simulink model "sim_linear_control_y"  (R2018a)
settings: Solver=ode3  StartTime=0.0  StopTime=20  FixedStep=0.001  RelTol=1e-3
values from neighbouring files (symbols this model uses):
  A = [-(Cf+Cr)/(m*Vx)  -(a*Cf-b*Cr)/(m*Vx)-Vx ... (first row only)    [lin_control_pos_v1.m]    (also in lin_control_y.m)
  B = [Cf/m; a*Cf/Iz]    [lin_control_pos_v1.m]    (also in lin_control_y.m)
  C = Col(3,:)    [lin_control_pos_v1.m]    (also in lin_control_y.m)
  CA = C*Aol    [lin_control_pos_v1.m]    (also in lin_control_y.m)
  g = 9.81    [lin_control_pos_v1.m]    (also in lin_control_y.m)
  intgA = zeros(2,2)    [lin_control_y.m]
  intgB = eye(2)    [lin_control_y.m]
  intgC = eye(2)    [lin_control_y.m]
  intgD = zeros(2,2)    [lin_control_y.m]
  invCB = pinv(C*Bol)    [lin_control_pos_v1.m]    (also in lin_control_y.m)
  K_ay = 8    [lin_control_pos_v1.m]    (also in lin_control_y.m = 4)
  K_v = 1    [lin_control_y.m]
  loop = 1    [lin_control_y.m]
  rho = 1/R    (= 0.05)    [lin_control_pos_v1.m]    (also in lin_control_y.m)
  Vx = 10/3.6    (= 2.77777777778)    [lin_control_pos_v1.m]    (also in lin_control_y.m)
  w = 10    [lin_control_pos_v1.m]    (also in lin_control_y.m)
settings Model: Creator=E183308  LastModifiedBy=E183308

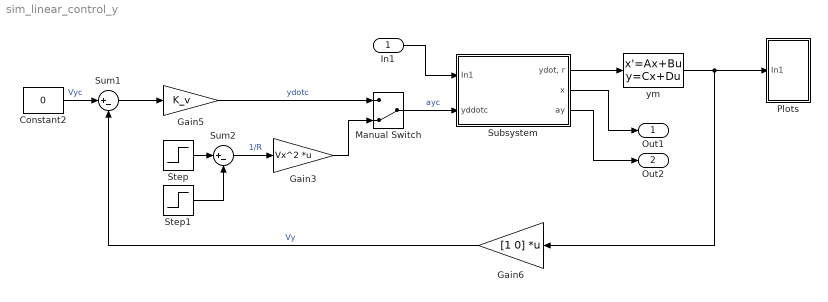
== system sim_linear_control_y ==
  In1 : Inport
  Constant2 : Constant  Value=0
  Gain3 : Gain  Gain=Vx^2  Multiplication=Matrix(K*u)
  Gain5 : Gain  Gain=K_v
  Gain6 : Gain  Gain=[1 0]  Multiplication=Matrix(K*u)
  Manual Switch : ManualSwitch  CurrentSetting=0
  Plots : Subsystem
  Step : Step  After=rho  SampleTime=0
  Step1 : Step  Time=10  After=rho  SampleTime=0
  Subsystem : Subsystem
  Sum1 : Sum  Inputs=|+-
  Sum2 : Sum  Inputs=|+-
  ym : StateSpace  A=intgA  B=intgB  C=intgC  D=intgD  InitialCondition=0
  Out1 : Outport
  Out2 : Outport  Port=2
  wires:
  Gain5/1 -> Manual Switch/1  "ydotc"
  Sum1/1 -> Gain5/1
  Gain6/1 -> Sum1/2  "Vy"
  In1/1 -> Subsystem/1(In1)
  Manual Switch/1 -> Subsystem/2(yddotc)  "ayc"
  ym/1 -> Gain6/1, Plots/1(In1)
  Subsystem/2(x) -> Out1/1
  Subsystem/1("ydot, r") -> ym/1
  Subsystem/3(ay) -> Out2/1
  Constant2/1 -> Sum1/1  "Vyc"
  Step1/1 -> Sum2/2
  Step/1 -> Sum2/1
  Sum2/1 -> Gain3/1  "1/R"
  Gain3/1 -> Manual Switch/2

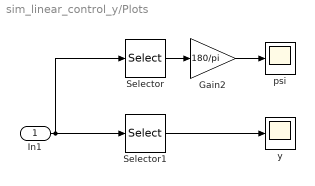
== system sim_linear_control_y/Plots ==
  In1 : Inport
  Gain2 : Gain  Gain=180/pi
  Selector : Selector  InputPortWidth=2  IndexOptions=Index vector (dialog)  Indices=2  OutputSizes=1
  Selector1 : Selector  InputPortWidth=2  IndexOptions=Index vector (dialog)  Indices=1  OutputSizes=1
  psi : Scope
  y : Scope
  wires:
  Gain2/1 -> psi/1
  In1/1 -> Selector1/1, Selector/1
  Selector/1 -> Gain2/1
  Selector1/1 -> y/1

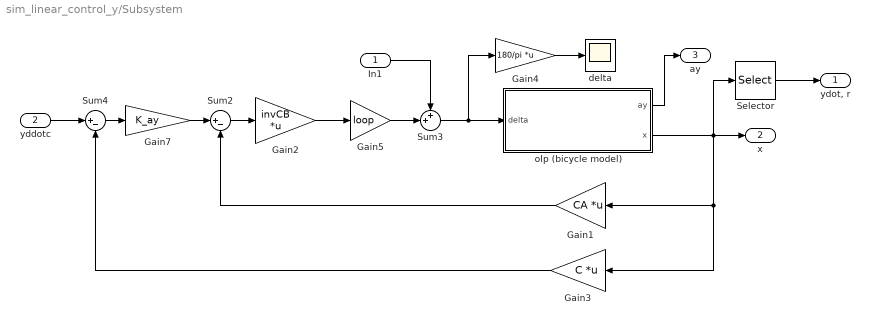
== system sim_linear_control_y/Subsystem ==
  In1 : Inport
  yddotc : Inport  Port=2
  Gain1 : Gain  Gain=CA  Multiplication=Matrix(K*u)
  Gain2 : Gain  Gain=invCB  Multiplication=Matrix(K*u)
  Gain3 : Gain  Gain=C  Multiplication=Matrix(K*u)
  Gain4 : Gain  Gain=180/pi  Multiplication=Matrix(K*u)
  Gain5 : Gain  Gain=loop
  Gain7 : Gain  Gain=K_ay
  Selector : Selector  InputPortWidth=3  IndexOptions=Index vector (dialog)  Indices=[1 2]  OutputSizes=1
  Sum2 : Sum  Inputs=|+-
  Sum3 : Sum  Inputs=++|
  Sum4 : Sum  Inputs=|+-
  delta : Scope
  olp (bicycle model) : Subsystem
  "ydot, r" : Outport
  x : Outport  Port=2
  ay : Outport  Port=3
  wires:
  Gain4/1 -> delta/1
  yddotc/1 -> Sum4/1
  Gain3/1 -> Sum4/2
  Gain2/1 -> Gain5/1
  Sum2/1 -> Gain2/1
  Sum4/1 -> Gain7/1
  Gain1/1 -> Sum2/2
  Gain7/1 -> Sum2/1
  olp (bicycle model)/2(x) -> Selector/1, Gain3/1, Gain1/1, x/1
  Selector/1 -> "ydot, r"/1
  Gain5/1 -> Sum3/2
  Sum3/1 -> Gain4/1, olp (bicycle model)/1(delta)
  In1/1 -> Sum3/1
  olp (bicycle model)/1(ay) -> ay/1

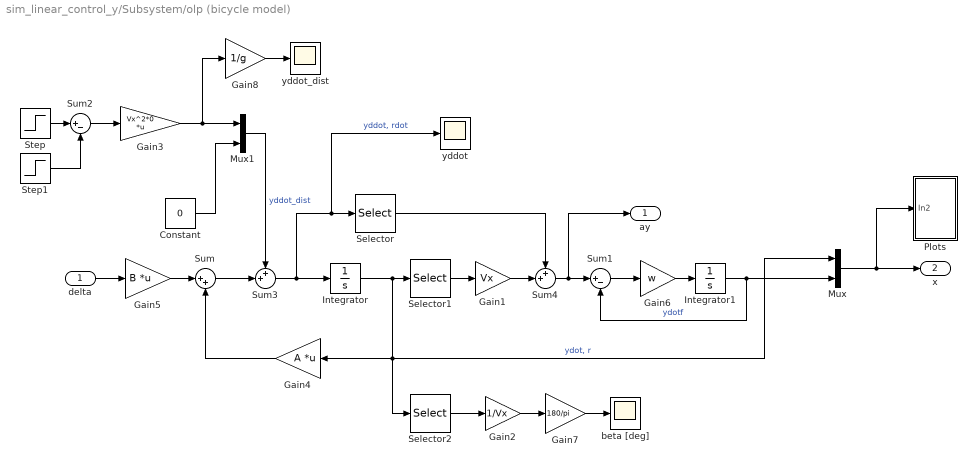
== system sim_linear_control_y/Subsystem/olp (bicycle model) ==
  delta : Inport
  Constant : Constant  Value=0
  Gain1 : Gain  Gain=Vx
  Gain2 : Gain  Gain=1/Vx
  Gain3 : Gain  Gain=Vx^2*0  Multiplication=Matrix(K*u)
  Gain4 : Gain  Gain=A  Multiplication=Matrix(K*u)
  Gain5 : Gain  Gain=B  Multiplication=Matrix(K*u)
  Gain6 : Gain  Gain=w
  Gain7 : Gain  Gain=180/pi
  Gain8 : Gain  Gain=1/g
  Integrator : Integrator  InitialCondition=[0;0]
  Integrator1 : Integrator
  Mux : Mux  Inputs=2
  Mux1 : Mux  Inputs=2
  Plots : Subsystem
  Selector : Selector  InputPortWidth=2  IndexOptions=Index vector (dialog)  Indices=1  OutputSizes=1
  Selector1 : Selector  InputPortWidth=2  IndexOptions=Index vector (dialog)  Indices=2  OutputSizes=1
  Selector2 : Selector  InputPortWidth=2  IndexOptions=Index vector (dialog)  Indices=1  OutputSizes=1
  Step : Step  After=rho  SampleTime=0
  Step1 : Step  Time=10  After=rho  SampleTime=0
  Sum : Sum  Inputs=|++
  Sum1 : Sum  Inputs=|+-
  Sum2 : Sum  Inputs=|+-
  Sum3 : Sum  Inputs=++|
  Sum4 : Sum  Inputs=++|
  beta [deg] : Scope
  yddot : Scope
  yddot_dist : Scope
  ay : Outport
  x : Outport  Port=2
  wires:
  Integrator/1 -> Selector1/1, Selector2/1, Gain4/1, Mux/1  "ydot, r"
  delta/1 -> Gain5/1
  Gain5/1 -> Sum/1
  Gain4/1 -> Sum/2
  Gain6/1 -> Integrator1/1
  Sum1/1 -> Gain6/1
  Mux/1 -> Plots/1(In2), x/1
  Integrator1/1 -> Sum1/2, Mux/2  "ydotf"
  Gain8/1 -> yddot_dist/1
  Sum2/1 -> Gain3/1
  Step/1 -> Sum2/1
  Step1/1 -> Sum2/2
  Sum/1 -> Sum3/2
  Sum3/1 -> yddot/1, Selector/1, Integrator/1  "yddot, rdot"
  Gain3/1 -> Mux1/1, Gain8/1
  Mux1/1 -> Sum3/1  "yddot_dist"
  Constant/1 -> Mux1/2
  Selector1/1 -> Gain1/1
  Gain1/1 -> Sum4/2
  Selector/1 -> Sum4/1
  Sum4/1 -> ay/1, Sum1/1
  Selector2/1 -> Gain2/1
  Gain2/1 -> Gain7/1
  Gain7/1 -> beta [deg]/1

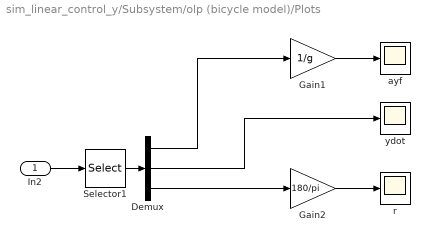
== system sim_linear_control_y/Subsystem/olp (bicycle model)/Plots ==
  In2 : Inport
  Demux : Demux  Outputs=3
  Gain1 : Gain  Gain=1/g
  Gain2 : Gain  Gain=180/pi
  Selector1 : Selector  InputPortWidth=3  IndexOptions=Index vector (dialog)  Indices=[3 1 2]  OutputSizes=1
  ayf : Scope
  r : Scope
  ydot : Scope
  wires:
  Demux/2 -> ydot/1
  Demux/3 -> Gain2/1
  Gain2/1 -> r/1
  In2/1 -> Selector1/1
  Demux/1 -> Gain1/1
  Selector1/1 -> Demux/1
  Gain1/1 -> ayf/1
